simulink model "monitor_ceder_S4"  (R2025b)
settings: Solver=VariableStepDiscrete  StartTime=0.0  StopTime=100  RelTol=1e-3
values from neighbouring files (symbols this model uses):
  m = mean(ts.Data(idx))    [barrido_S0.m]
  nPMU = 5    [barrido_S4.m]
undefined symbols (not defined in the file or in its folder): n, periodGen, ratePQ
settings Model: Creator=ildio  LastModifiedBy=ildio

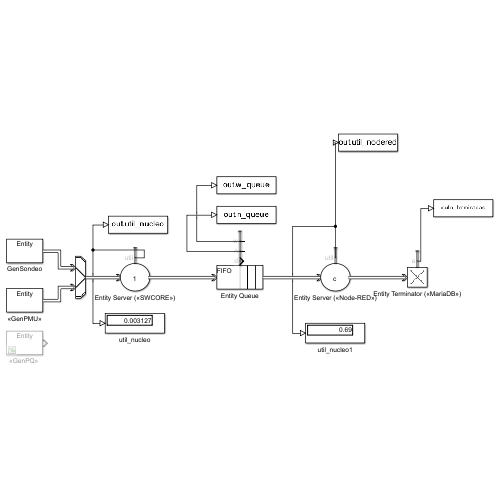
[thumbnail: Simulink's stored preview of the top-level diagram]
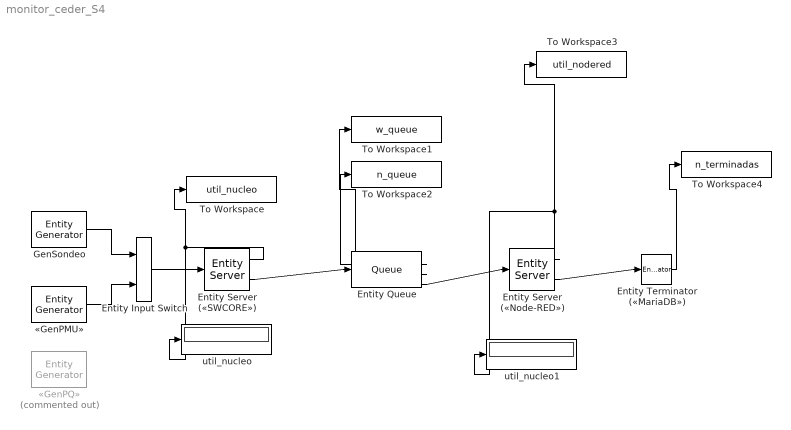
== system monitor_ceder_S4 ==
  Entity Input Switch : EntityInputSwitch  InputPortMessageModes=m,m  OutputPortMessageModes=m
  Entity Queue : Queue  InputPortMessageModes=m  OutputPortMessageModes=n,n,n,m  Capacity=100  NumberEntitiesDeparted=on  NumberEntitiesInBlock=on  AverageWait=on
      settings: OutputPortMap=o0,o1,o2,o5
  Entity Server («Node-RED») : EntityServer  InputPortMessageModes=m  OutputPortMessageModes=n,m  Capacity=c  ServiceTimeValue=tResp  ServiceTimeAction=dt = -tResp .* log(rand(size(entitySys.id)));  Utilization=on
      settings: OutputPortMap=o5,o9
  Entity Server («SWCORE») : EntityServer  InputPortMessageModes=m  OutputPortMessageModes=n,m  Capacity=1  ServiceTimeSource=MATLAB action  ServiceTimeValue=tNucleo  ServiceTimeAction=dt = entity.Lbytes * 8 / Cenlace;  Utilization=on
      settings: OutputPortMap=o5,o9
  Entity Terminator («MariaDB») : EntityTerminator  InputPortMessageModes=m  NumberEntitiesArrived=on
      settings: OutputPortMap=o0
  GenSondeo : EntityGenerator  OutputPortMessageModes=m  Period=periodGen  AttributeName=Attribute1|Lbytes  AttributeInitialValue=1|86  EntityType=Structured  EntityTypeName=Entity
  To Workspace : ToWorkspace  VariableName=util_nucleo  SaveFormat=Timeseries  SampleTime=-1
      settings: Decimation=3
  To Workspace1 : ToWorkspace  VariableName=w_queue  SaveFormat=Timeseries  SampleTime=-1
      settings: Decimation=3
  To Workspace2 : ToWorkspace  VariableName=n_queue  SaveFormat=Timeseries  SampleTime=-1
      settings: Decimation=3
  To Workspace3 : ToWorkspace  VariableName=util_nodered  SaveFormat=Timeseries  SampleTime=-1
      settings: Decimation=3
  To Workspace4 : ToWorkspace  VariableName=n_terminadas  SaveFormat=Timeseries  SampleTime=-1
      settings: Decimation=3
  util_nucleo : Display
  util_nucleo1 : Display
  «GenPMU» : EntityGenerator  OutputPortMessageModes=m  Period=1/(nPMU*50)  IntergenerationTimeAction=dt = entity.Lbytes * 8 / Cenlace;  AttributeName=Attribute1|Lbytes  AttributeInitialValue=1|110  EntityType=Structured  EntityTypeName=Entity
  "«GenPQ» " : EntityGenerator  Commented=on  OutputPortMessageModes=m  Period=1/(15*ratePQ)  IntergenerationTimeAction=dt = entity.Lbytes * 8 / Cenlace;  AttributeName=Attribute1|Lbytes  AttributeInitialValue=1|Lpq  EntityType=Structured  EntityTypeName=Entity
  wires:
  Entity Server («Node-RED»)/2 -> Entity Terminator («MariaDB»)/1
  Entity Queue/4 -> Entity Server («Node-RED»)/1
  Entity Server («SWCORE»)/2 -> Entity Queue/1
  Entity Server («SWCORE»)/1 -> util_nucleo/1, To Workspace/1
  Entity Server («Node-RED»)/1 -> To Workspace3/1, util_nucleo1/1
  Entity Queue/3 -> To Workspace1/1
  Entity Queue/2 -> To Workspace2/1
  Entity Terminator («MariaDB»)/1 -> To Workspace4/1
  GenSondeo/1 -> Entity Input Switch/1
  Entity Input Switch/1 -> Entity Server («SWCORE»)/1
  «GenPMU»/1 -> Entity Input Switch/2
